simulink model "Drv_Unit"  (R2020b)
settings: configuration reference "gen_config" (kept outside this file)
libraries: simulink_extras x1
settings Model: DataDictionary=Hybrid_vehicle.sldd  SimulationMode=accelerator  OrderedModelArguments=off  Creator=Georg  LastModifiedBy=jy
settings ConfigSetRef: SourceName=gen_config

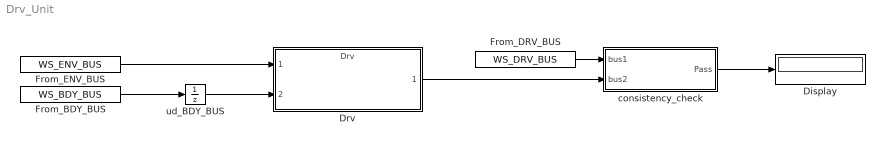
== system Drv_Unit ==
  Display : Display
  Drv : ModelReference  ModelNameDialog=Drv  SimulationMode=Normal  ModelReferenceVersion=2.22
  From_BDY_BUS : FromWorkspace  VariableName=WS_BDY_BUS  OutDataTypeStr=Bus: BDY_BUS  SampleTime=-1  Interpolate=off  OutputAfterFinalValue=Holding final value
  From_DRV_BUS : FromWorkspace  VariableName=WS_DRV_BUS  OutDataTypeStr=Bus: DRV_BUS  SampleTime=-1  Interpolate=off  OutputAfterFinalValue=Holding final value
  From_ENV_BUS : FromWorkspace  VariableName=WS_ENV_BUS  OutDataTypeStr=Bus: ENV_BUS  SampleTime=-1  Interpolate=off  OutputAfterFinalValue=Holding final value
  consistency_check : Subsystem
  ud_BDY_BUS : UnitDelay  SampleTime=-1  HasFrameUpgradeWarning=on
  wires:
  From_ENV_BUS/1 -> Drv/1
  From_BDY_BUS/1 -> ud_BDY_BUS/1
  ud_BDY_BUS/1 -> Drv/2
  From_DRV_BUS/1 -> consistency_check/1(bus1)
  Drv/1 -> consistency_check/2(bus2)
  consistency_check/1(Pass) -> Display/1

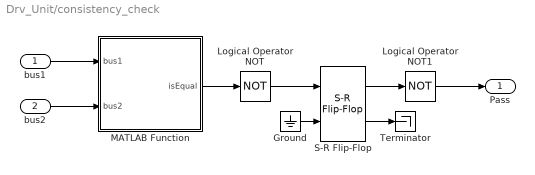
== system Drv_Unit/consistency_check ==
  bus1 : Inport
  bus2 : Inport  Port=2
  Ground : Ground
  Logical Operator NOT : Logic  Operator=NOT  AllPortsSameDT=off  OutDataTypeStr=boolean
  Logical Operator NOT1 : Logic  Operator=NOT  AllPortsSameDT=off  OutDataTypeStr=boolean
  MATLAB Function : MATLAB Function  TreatAsAtomicUnit=on
  S-R Flip-Flop : simulink_extras/Flip Flops/S-R Flip-Flop  initial_condition=0
  Terminator : Terminator
  Pass : Outport
  wires:
  bus1/1 -> MATLAB Function/1(bus1)
  bus2/1 -> MATLAB Function/2(bus2)
  MATLAB Function/1(isEqual) -> Logical Operator NOT/1
  Logical Operator NOT/1 -> S-R Flip-Flop/1
  Ground/1 -> S-R Flip-Flop/2
  S-R Flip-Flop/2 -> Terminator/1
  S-R Flip-Flop/1 -> Logical Operator NOT1/1
  Logical Operator NOT1/1 -> Pass/1

== matlab function Drv_Unit/consistency_check/MATLAB Function ==
  data: bus1 input; isEqual output; bus2 input
function isEqual = fcn(bus1, bus2)
isEqual = isequal(bus1, bus2);
